simulink library "Dynamic_2D_Lookup_Table"  (R2018b)
settings: Solver=ode45  StartTime=0.0  StopTime=10.0  RelTol=1e-3  EnableMultiTasking=on
settings Model: Creator=agupte  LastModifiedBy=James Reed
settings DataIOCC: LimitDataPoints=on  SaveFormat=Array  SignalLoggingSaveFormat=ModelDataLogs
settings OptimizationCC: ExpressionDepthLimit=2147483647  LifeSpan=inf
settings DebuggingCC: UnderspecifiedInitializationDetection=Classic  MergeDetectMultiDrivingBlocksExec=none  SolverPrmCheckMsg=warning  FcnCallInpInsideContextMsg=warning  StateNameClashWarn=warning  SFUnexpectedBacktrackingDiag=warning  SFNoUnconditionalDefaultTransitionDiag=warning  SFExecutionAtInitializationDiag=none
settings HardwareCC: ProdBitPerPointer=32  ProdBitPerSizeT=32  ProdBitPerPtrDiffT=32  ProdLargestAtomicFloat=None  ProdIntDivRoundTo=Undefined  ProdEndianess=Unspecified  ProdWordSize=32  ProdHWDeviceType=32-bit Generic
settings ModelReferenceCC: PropagateSignalLabelsOutOfModel=off
settings SFSimCC: SimUseLocalCustomCode=off
settings RTWCC: RTWUseLocalCustomCode=off
settings CodeAppCC: StateflowObjectComments=on
settings GRTTargetCC: TargetLangStandard=C89/C90 (ANSI)  GeneratePreprocessorConditionals=Disable all  CombineOutputUpdateFcns=off  GRTInterface=on
settings ConfigComp: CovMetricSettings=dw  CovHtmlReporting=on  CovSaveCumulativeToWorkspaceVar=on  CovSaveSingleToWorkspaceVar=on  CovExternalEMLEnable=off

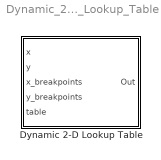
== system Dynamic_2D_Lookup_Table ==
  Dynamic 2-D Lookup Table : Subsystem  mask(Dynamic 2-D Look-up Table){}
      mask help:
      | Inputs should be in the following format:
      | 1. x: Scalar x-coordinate
      | 2. y: Scalar y-coordinate
      | 3: x_breakpoints: Monotonically increasing vector of breakpoints for x-data
      | 4: y_breakpoints: Monotonically increasing vector of breakpoints for y-data
      | 5. table: Tabular data. Number of rows and columns in table should match the length of the breakpoints vector.

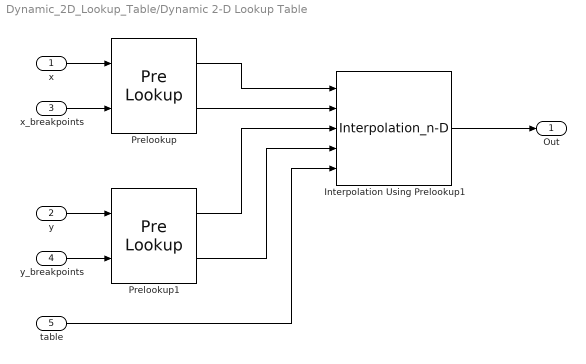
== system Dynamic_2D_Lookup_Table/Dynamic 2-D Lookup Table ==
  x : Inport
  y : Inport  Port=2
  x_breakpoints : Inport  Port=3
  y_breakpoints : Inport  Port=4
  table : Inport  Port=5
  Interpolation Using Prelookup1 : Interpolation_n-D  TableSource=Input port
      settings: InputPortMap=u0,u1,u2,u3,p2
  Prelookup : PreLookup  BreakpointsDataSource=Input port  BreakpointsData=[1:4]  FractionDataTypeStr=double
      settings: InputPortMap=u0,p1
  Prelookup1 : PreLookup  BreakpointsDataSource=Input port  BreakpointsData=[1:4]  FractionDataTypeStr=double
      settings: InputPortMap=u0,p1
  Out : Outport
  wires:
  x/1 -> Prelookup/1
  Interpolation Using Prelookup1/1 -> Out/1
  table/1 -> Interpolation Using Prelookup1/5
  y/1 -> Prelookup1/1
  x_breakpoints/1 -> Prelookup/2
  y_breakpoints/1 -> Prelookup1/2
  Prelookup/2 -> Interpolation Using Prelookup1/2
  Prelookup/1 -> Interpolation Using Prelookup1/1
  Prelookup1/2 -> Interpolation Using Prelookup1/4
  Prelookup1/1 -> Interpolation Using Prelookup1/3
